simulink model "sineWaveProject"  (R2022a)
settings: Solver=VariableStepAuto  StartTime=0.0  StopTime=10.0  RelTol=1e-3
settings Model: Creator=Waleed  LastModifiedBy=Waleed

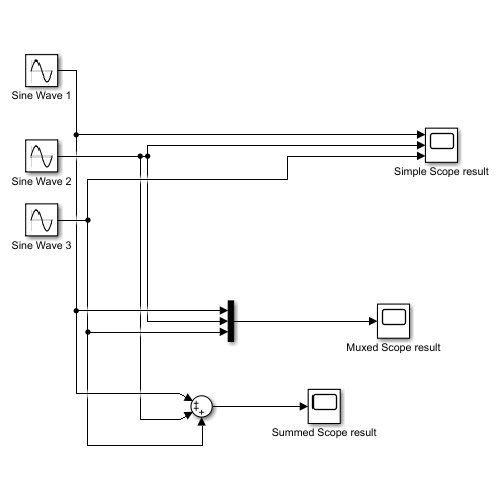
[thumbnail: Simulink's stored preview of the top-level diagram]
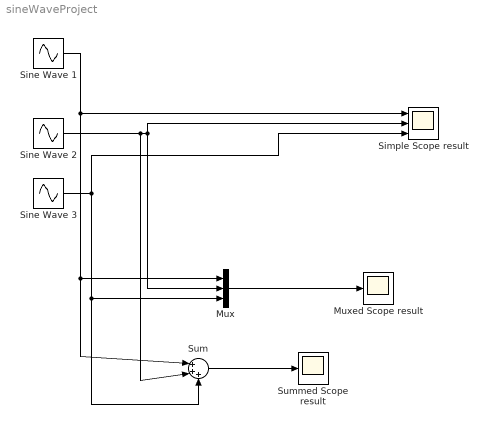
== system sineWaveProject ==
  Mux : Mux  Inputs=3
  Muxed Scope result : Scope
  Simple Scope result : Scope  NumInputPorts=3
  Sine Wave 1 : Sin  SampleTime=0
  Sine Wave 2 : Sin  Amplitude=2  Frequency=10  SampleTime=0
  Sine Wave 3 : Sin  Amplitude=0.5  Frequency=5  SampleTime=0
  Sum : Sum  Inputs=|+++
  Summed Scope result : Scope
  wires:
  Sine Wave 1/1 -> Sum/1, Mux/1, Simple Scope result/1
  Sine Wave 2/1 -> Sum/2, Mux/2, Simple Scope result/2
  Sine Wave 3/1 -> Sum/3, Mux/3, Simple Scope result/3
  Mux/1 -> Muxed Scope result/1
  Sum/1 -> Summed Scope result/1
